simulink library "BupSimulinkLibraries"  (R2018a)
settings: Solver=VariableStepAuto  StartTime=0.0  StopTime=10.0  RelTol=1e-3
settings Model: Creator=User33  LastModifiedBy=User33

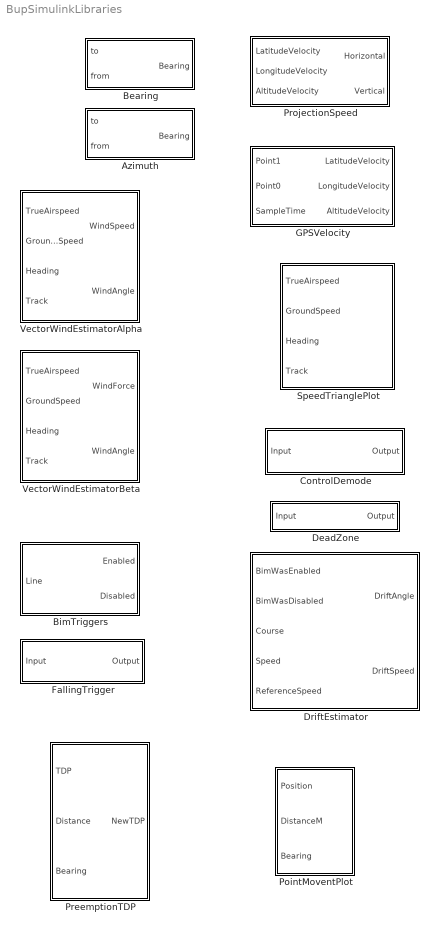
== system BupSimulinkLibraries ==
  Azimuth : Subsystem  TreatAsAtomicUnit=on
  Bearing : Subsystem  TreatAsAtomicUnit=on
  BimTriggers : Subsystem
  ControlDemode : Subsystem
  DeadZone : Subsystem
  DriftEstimator : Stateflow chart  TreatAsAtomicUnit=on
  FallingTrigger : Subsystem
  GPSVelocity : Subsystem  TreatAsAtomicUnit=on
  PointMoventPlot : Subsystem
  PreemptionTDP : Subsystem
  ProjectionSpeed : Subsystem  TreatAsAtomicUnit=on
  SpeedTrianglePlot : Subsystem
  VectorWindEstimatorAlpha : Subsystem  TreatAsAtomicUnit=on
      mask Display: image('500px-Drift_1.png');
  VectorWindEstimatorBeta : Subsystem  TreatAsAtomicUnit=on
      mask Display: image('500px-Drift_1.png');

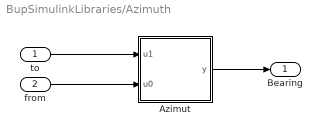
== system BupSimulinkLibraries/Azimuth ==
  to : Inport
  from : Inport  Port=2
  Azimut : MATLAB Function  TreatAsAtomicUnit=on
  Bearing : Outport
  wires:
  to/1 -> Azimut/1(u1)
  from/1 -> Azimut/2(u0)
  Azimut/1(y) -> Bearing/1

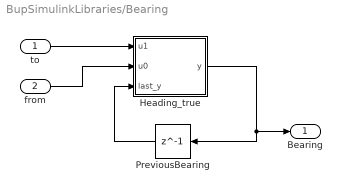
== system BupSimulinkLibraries/Bearing ==
  to : Inport
  from : Inport  Port=2
  Heading_true : MATLAB Function  TreatAsAtomicUnit=on
  PreviousBearing : Delay  DelayLength=1  InitialCondition=0
  Bearing : Outport
  wires:
  to/1 -> Heading_true/1(u1)
  Heading_true/1(y) -> PreviousBearing/1, Bearing/1
  from/1 -> Heading_true/2(u0)
  PreviousBearing/1 -> Heading_true/3(last_y)

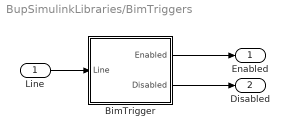
== system BupSimulinkLibraries/BimTriggers ==
  Line : Inport
  BimTrigger : Stateflow chart  TreatAsAtomicUnit=on
  Enabled : Outport
  Disabled : Outport  Port=2
  wires:
  Line/1 -> BimTrigger/1(Line)
  BimTrigger/1(Enabled) -> Enabled/1
  BimTrigger/2(Disabled) -> Disabled/1

== system BupSimulinkLibraries/ControlDemode ==
  Input : Inport
  ControlDemode : MATLAB Function  TreatAsAtomicUnit=on
  Output : Outport
  wires:
  ControlDemode/1(y) -> Output/1
  Input/1 -> ControlDemode/1(u)

== system BupSimulinkLibraries/DeadZone ==
  Input : Inport
  DeadZone : MATLAB Function  TreatAsAtomicUnit=on
  Output : Outport
  wires:
  DeadZone/1(y) -> Output/1
  Input/1 -> DeadZone/1(u)

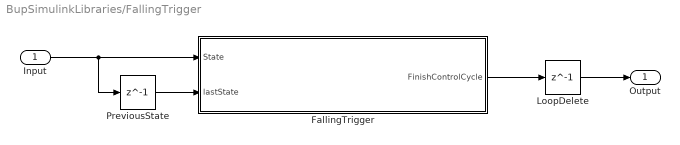
== system BupSimulinkLibraries/FallingTrigger ==
  Input : Inport
  FallingTrigger : MATLAB Function  TreatAsAtomicUnit=on
  LoopDelete : Delay  DelayLength=1
  PreviousState : Delay  DelayLength=1
  Output : Outport
  wires:
  FallingTrigger/1(FinishControlCycle) -> LoopDelete/1
  Input/1 -> PreviousState/1, FallingTrigger/1(State)
  LoopDelete/1 -> Output/1
  PreviousState/1 -> FallingTrigger/2(lastState)

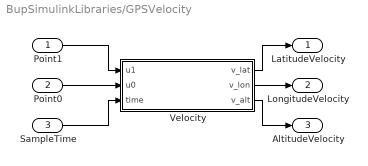
== system BupSimulinkLibraries/GPSVelocity ==
  Point1 : Inport
  Point0 : Inport  Port=2
  SampleTime : Inport  Port=3
  Velocity : MATLAB Function  TreatAsAtomicUnit=on
  LatitudeVelocity : Outport
  LongitudeVelocity : Outport  Port=2
  AltitudeVelocity : Outport  Port=3
  wires:
  Velocity/1(v_lat) -> LatitudeVelocity/1
  Point0/1 -> Velocity/2(u0)
  Point1/1 -> Velocity/1(u1)
  Velocity/3(v_alt) -> AltitudeVelocity/1
  Velocity/2(v_lon) -> LongitudeVelocity/1
  SampleTime/1 -> Velocity/3(time)

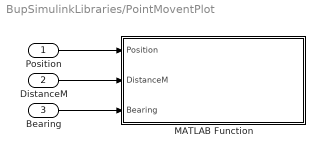
== system BupSimulinkLibraries/PointMoventPlot ==
  Position : Inport
  DistanceM : Inport  Port=2
  Bearing : Inport  Port=3
  MATLAB Function : MATLAB Function  TreatAsAtomicUnit=on
  wires:
  DistanceM/1 -> MATLAB Function/2(DistanceM)
  Bearing/1 -> MATLAB Function/3(Bearing)
  Position/1 -> MATLAB Function/1(Position)

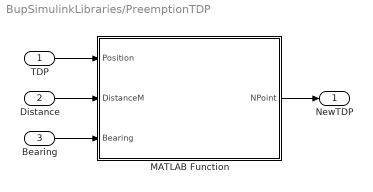
== system BupSimulinkLibraries/PreemptionTDP ==
  TDP : Inport
  Distance : Inport  Port=2
  Bearing : Inport  Port=3
  MATLAB Function : MATLAB Function  TreatAsAtomicUnit=on
  NewTDP : Outport
  wires:
  Bearing/1 -> MATLAB Function/3(Bearing)
  MATLAB Function/1(NPoint) -> NewTDP/1
  TDP/1 -> MATLAB Function/1(Position)
  Distance/1 -> MATLAB Function/2(DistanceM)

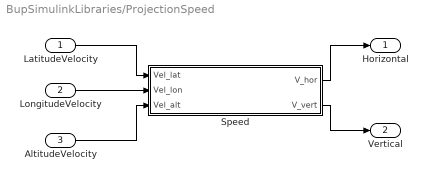
== system BupSimulinkLibraries/ProjectionSpeed ==
  LatitudeVelocity : Inport
  LongitudeVelocity : Inport  Port=2
  AltitudeVelocity : Inport  Port=3
  Speed : MATLAB Function  TreatAsAtomicUnit=on
  Horizontal : Outport
  Vertical : Outport  Port=2
  wires:
  LatitudeVelocity/1 -> Speed/1(Vel_lat)
  Speed/1(V_hor) -> Horizontal/1
  LongitudeVelocity/1 -> Speed/2(Vel_lon)
  AltitudeVelocity/1 -> Speed/3(Vel_alt)
  Speed/2(V_vert) -> Vertical/1

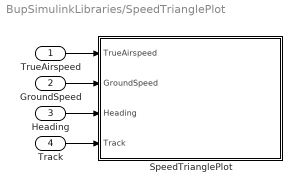
== system BupSimulinkLibraries/SpeedTrianglePlot ==
  TrueAirspeed : Inport
  GroundSpeed : Inport  Port=2
  Heading : Inport  Port=3
  Track : Inport  Port=4
  SpeedTrianglePlot : MATLAB Function  TreatAsAtomicUnit=on
  wires:
  Track/1 -> SpeedTrianglePlot/4(Track)
  Heading/1 -> SpeedTrianglePlot/3(Heading)
  GroundSpeed/1 -> SpeedTrianglePlot/2(GroundSpeed)
  TrueAirspeed/1 -> SpeedTrianglePlot/1(TrueAirspeed)

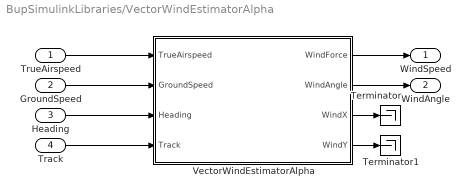
== system BupSimulinkLibraries/VectorWindEstimatorAlpha ==
  TrueAirspeed : Inport
  GroundSpeed : Inport  Port=2
  Heading : Inport  Port=3
  Track : Inport  Port=4
  Terminator : Terminator
  Terminator1 : Terminator
  VectorWindEstimatorAlpha : MATLAB Function  TreatAsAtomicUnit=on
  WindSpeed : Outport
  WindAngle : Outport  Port=2
  wires:
  VectorWindEstimatorAlpha/3(WindX) -> Terminator/1
  GroundSpeed/1 -> VectorWindEstimatorAlpha/2(GroundSpeed)
  Heading/1 -> VectorWindEstimatorAlpha/3(Heading)
  VectorWindEstimatorAlpha/1(WindForce) -> WindSpeed/1
  TrueAirspeed/1 -> VectorWindEstimatorAlpha/1(TrueAirspeed)
  Track/1 -> VectorWindEstimatorAlpha/4(Track)
  VectorWindEstimatorAlpha/4(WindY) -> Terminator1/1
  VectorWindEstimatorAlpha/2(WindAngle) -> WindAngle/1

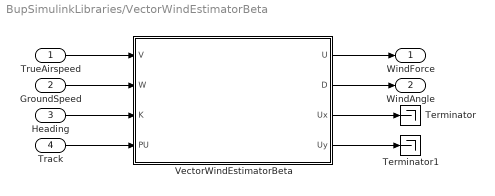
== system BupSimulinkLibraries/VectorWindEstimatorBeta ==
  TrueAirspeed : Inport
  GroundSpeed : Inport  Port=2
  Heading : Inport  Port=3
  Track : Inport  Port=4
  Terminator : Terminator
  Terminator1 : Terminator
  VectorWindEstimatorBeta : MATLAB Function  TreatAsAtomicUnit=on
  WindForce : Outport
  WindAngle : Outport  Port=2
  wires:
  VectorWindEstimatorBeta/2(D) -> WindAngle/1
  VectorWindEstimatorBeta/4(Uy) -> Terminator1/1
  VectorWindEstimatorBeta/1(U) -> WindForce/1
  Track/1 -> VectorWindEstimatorBeta/4(PU)
  Heading/1 -> VectorWindEstimatorBeta/3(K)
  GroundSpeed/1 -> VectorWindEstimatorBeta/2(W)
  VectorWindEstimatorBeta/3(Ux) -> Terminator/1
  TrueAirspeed/1 -> VectorWindEstimatorBeta/1(V)

== matlab function BupSimulinkLibraries/SpeedTrianglePlot/SpeedTrianglePlot ==
  data: TrueAirspeed input size=1; GroundSpeed input size=1; Heading input size=1; Track input size=1
%%%%%%%%%%%%%%%%%%%%%%%%%%%%%%%%%%%%%%%%%%%%%%%%%%%%%%%%%%%%%%%%%%%%%%%%%%%
%
%   Расчет и построение навигационного треугольника скоростей
%
%   Обозначения:
%   TrueAirspeed - Истинная воздушная скорость
%   GroundSpeed - Скорость относительно земли
%   Heading - Направление продольной оси
%   Track - Путевой курс
%%%%%%%%%%%%%%%%%%%%%%%%%%%%%%%%%%%%%%%%%%%%%%%%%%%%%%%%%%%%%%%%%%%%%%%%%%%
function SpeedTrianglePlot(TrueAirspeed, GroundSpeed, Heading, Track)
    %% Определяем проекции вектора воздушной скорости
    TrueAirspeedX = TrueAirspeed * cos(pi/2 - Heading);
    TrueAirspeedY = TrueAirspeed * cos(- Heading);
    %% Определяем проекции вектора путевой скорости
    GroundSpeedX = GroundSpeed * cos(pi/2 - Track);
    GroundSpeedY = GroundSpeed * cos(- Track);
    %% Определяем проекции вектора ветра
    WindX = -(TrueAirspeedX - GroundSpeedX);
    WindY = -(TrueAirspeedY - GroundSpeedY);
    %% Визуализация
    figure(55)
    plot([0 TrueAirspeedX], [0 TrueAirspeedY]);
    hold on
    plot([0 GroundSpeedX], [0 GroundSpeedY]);
    hold on
    plot([TrueAirspeedX TrueAirspeedX+WindX], [TrueAirspeedY TrueAirspeedY+WindY]);
    grid on
    hold off
    axis([-30 +30 -30 +30])
end

== matlab function BupSimulinkLibraries/Azimuth/Azimut ==
  data: u1 input size=3; u0 input size=3; y output size=1
function y = fcn(u1, u0)
% u0 - точка отсчета
% u1 - конечная точка
% la - долгота
% fi - широта
la1 = u0(2)*pi/180;
fi1 = u0(1)*pi/180;
la2 = u1(2)*pi/180;
fi2 = u1(1)*pi/180;
delta_la = la2-la1;
y = atan2(sin(delta_la)*cos(fi2), cos(fi1)*sin(fi2)-sin(fi1)*cos(fi2)*cos(delta_la));
y = rem((y + 2*pi), 2*pi);
end

== matlab function BupSimulinkLibraries/Bearing/Heading_true ==
  data: u1 input size=3; u0 input size=3; y output size=1; last_y input size=1
function y = fcn(u1, u0, last_y)
%% Высчитаем, как изменились координаты
un = u1 - u0;
d_lat = un(1);
d_lon = un(2);
%% Условие для определения кратчайшего пути с учетом переходов между
% меридианами 0 и 180 по долготе
if d_lon > 180
    d_lon = d_lon - 360;
elseif d_lon < (-180)
        d_lon = d_lon +360;
end
%% Расчет курса
un_pow1 = d_lat*d_lat;
un_pow2 = d_lon*d_lon;
if (un_pow1 < 1e-16) && (un_pow2 < 1e-16)
    y = last_y;
else
    x = acos( d_lon / (sqrt(un_pow2 + un_pow1)));
    y = acos( d_lat / (sqrt(un_pow2 + un_pow1)));
    if x > pi/2
        y = 2*pi - y;
    end
end

== matlab function BupSimulinkLibraries/ControlDemode/ControlDemode ==
  data: u input size=1; y output size=1
function y = ControlDemode(u)
    % Здесь переводим угол из диапазона [0 360]
    % в диапазон [-180 180], что позволит нам определять
    % оптимальное направление разворота (лево и право)
    y = u;
    % Если больше 180
    if y > pi
        % то это уже отрицательная полуокружность
        y = y - 2*pi;
    % Если меньше -180
    elseif (y < (-pi))
        % то это уже положительная полуокружность
        y = y + 2*pi;
    end
end

== matlab function BupSimulinkLibraries/GPSVelocity/Velocity ==
  data: u1 input size=3; v_lat output size=1; u0 input size=3; v_lon output size=1; v_alt output size=1; time input size=1
%%%%%%%%%%%%%%%%%%%%%%%%%%%%%%%%%%%%%%%%%%%%%%%%%%%%%%%%%%%%%%%%%%%%%%%%%%%
%
%   GPSPos2Speed - Определение скорости по сигналам GPS
%   u1 - Точка относительно, которой считаем перемещение (lat, lon, alt)
%   u0 - Точка до которой отладываем перемещение (lat, lon, alt)
%   time - Время между замерами координат
%
%%%%%%%%%%%%%%%%%%%%%%%%%%%%%%%%%%%%%%%%%%%%%%%%%%%%%%%%%%%%%%%%%%%%%%%%%%%
function [v_lat, v_lon, v_alt] = GPSPos2Speed(u1, u0, time)
    un = u1-u0;
    v_lat = un(1)*40000/360*1000/time;
    v_lon = un(2)*(40000/360*1000/time * cos(pi/180*u0(1)));
    v_alt = un(3);
end

== matlab function BupSimulinkLibraries/DeadZone/DeadZone ==
  data: u input size=1; y output size=1
%%%%%%%%%%%%%%%%%%%%%%%%%%%%%%%%%%%%%%%%%%%%%%%%%%%%%%%%%%%%%%%%%%%%%%%%%%%
%
%   Звено нечувствительности
%
%%%%%%%%%%%%%%%%%%%%%%%%%%%%%%%%%%%%%%%%%%%%%%%%%%%%%%%%%%%%%%%%%%%%%%%%%%%
function y = DeadZone(u)
if abs(u) < 20
    y = 0;
else
    y = u;
end
% if u > 10
%     y = 50;
% elseif u < - 10
%     y = -50;
% else
%     y = 0;
% end

== matlab function BupSimulinkLibraries/FallingTrigger/FallingTrigger ==
  data: State input size=1; FinishControlCycle output boolean size=1; lastState input size=1
function FinishControlCycle = FallingTrigger(State, lastState)
    if lastState > 0 && State <= 0
        FinishControlCycle = true;

    elseif lastState < 0 && State >= 0
        FinishControlCycle = true;

    else 
        FinishControlCycle = false;
    end
end

== matlab function BupSimulinkLibraries/ProjectionSpeed/Speed ==
  data: Vel_lat input size=1; V_hor output size=1; Vel_lon input size=1; Vel_alt input size=1; V_vert output size=1
%%%%%%%%%%%%%%%%%%%%%%%%%%%%%%%%%%%%%%%%%%%%%%%%%%%%%%%%%%%%%%%%%%%%%%%%%%%
%
%   SpeedProjections - Пересчет проекций векторов скорости по lat, lon, alt
%   в горизонтальную и вертикальную скорость полёта
%
%%%%%%%%%%%%%%%%%%%%%%%%%%%%%%%%%%%%%%%%%%%%%%%%%%%%%%%%%%%%%%%%%%%%%%%%%%%
function [V_hor, V_vert] = SpeedProjections(Vel_lat, Vel_lon, Vel_alt)
    V_hor = sqrt(Vel_lat^2 + Vel_lon^2);
    V_vert = abs(Vel_alt);
end

== stateflow chart BupSimulinkLibraries/BimTriggers/BimTrigger ==
  state Triggers
    state DisabledTrigger [parallel]
      if LastLineState > 0 && Line <=0
      Disabled = true;
      elseif LastLineState < 0 && Line >=0
      Disabled = true;
      else
      Disabled = false;
      end
      settings: executionOrder=1
    state EnabledTrigger1 [parallel]
      if LastLineState == 0 && Line > 0
      Enabled = true;
      elseif LastLineState == 0 && Line < 0
      Enabled = true;
      else
      Enabled = false;
      end
      settings: executionOrder=2
    state RemeberLastState [parallel]
      LastLineState = Line;
      settings: executionOrder=3
  data: Enabled output boolean size=1; Disabled output boolean size=1; LastLineState local double size=1 =0; Line input double size=1

== stateflow chart BupSimulinkLibraries/DriftEstimator ==
  state FixBeforeCorrection
    exit:
    RealCourse = Course;
    RealSpeed  = Speed;
  state FixAfterCorrection
    exit:
    ReferenceCourse = Course;
  state DriftSolver
    [DriftSpeed, DriftAngle] = SpeedTriangle(ReferenceSpeed, RealSpeed, ReferenceCourse, RealCourse);
    %SpeedTrianglePlot(ReferenceSpeed, RealSpeed, ReferenceCourse, RealCourse);
  (default) -> FixAfterCorrection
  FixAfterCorrection -> FixBeforeCorrection : [BimWasDisabled == 1]
  DriftSolver -> FixAfterCorrection
  FixBeforeCorrection -> DriftSolver : [BimWasEnabled == 1]
  data: BimWasEnabled input boolean size=1; BimWasDisabled input boolean size=1; Course input double size=1; Speed input double size=1; DriftAngle output double size=1; DriftSpeed output double size=1; ReferenceCourse local double size=1; RealSpeed local double size=1; RealCourse local double size=1; ReferenceSpeed input double size=1

== matlab function BupSimulinkLibraries/PreemptionTDP/MATLAB Function ==
  data: Position input double size=3; NPoint output double size=[1 3]; DistanceM input double size=1; Bearing input double size=1
%%%%%%%%%%%%%%%%%%%%%%%%%%%%%%%%%%%%%%%%%%%%%%%%%%%%%%%%%%%%%%%%%%%%%%%%%%%
%
%   PointMovement - Перемещение из точки Position на расстояние 
%   DistanceM (метры) в направлении относительно севера Bearing
%
%%%%%%%%%%%%%%%%%%%%%%%%%%%%%%%%%%%%%%%%%%%%%%%%%%%%%%%%%%%%%%%%%%%%%%%%%%%
function NPoint = PointMovement(Position, DistanceM, Bearing)
    %% Рассчитаем угловое расстояние
    AngularDistance = DistanceM/6378160;
    %% Координаты в радианы
    Lat1 = Position(1)/180*pi;
    Lon1 = Position(2)/180*pi;
    %% Получаем координаты точки перемещения
    Lat2 = asin(sin(Lat1)*cos(AngularDistance) + cos(Lat1)*sin(AngularDistance)*cos(Bearing));
    Lon2 = Lon1 + atan2(sin(Bearing)*sin(AngularDistance)*cos(Lat1), cos(AngularDistance)-sin(Lat1)*sin(Lat2));
    %% Переводим в градусы
    Lat2 = Lat2/pi*180;
    Lon2 = Lon2/pi*180;
    NPoint = [Lat2, Lon2, Position(3)];
end

== matlab function BupSimulinkLibraries/PointMoventPlot/MATLAB Function ==
  data: Position input double size=3; DistanceM input double size=1; Bearing input double size=1
%%%%%%%%%%%%%%%%%%%%%%%%%%%%%%%%%%%%%%%%%%%%%%%%%%%%%%%%%%%%%%%%%%%%%%%%%%%
%
%   PointMovementPlot - Отрисовка перемещения из точки Position на 
%   расстояние DistanceM (метры) в направлении относительно севера Bearing
%
%%%%%%%%%%%%%%%%%%%%%%%%%%%%%%%%%%%%%%%%%%%%%%%%%%%%%%%%%%%%%%%%%%%%%%%%%%%
function PointMovementPlot(Position, DistanceM, Bearing)
    %% Рассчитаем угловое расстояние
    AngularDistance = DistanceM/6378160;
    %% Координаты в радианы
    Lat1 = Position(1)/180*pi;
    Lon1 = Position(2)/180*pi;
    %% Получаем координаты точки перемещения
    Lat2 = asin(sin(Lat1)*cos(AngularDistance) + cos(Lat1)*sin(AngularDistance)*cos(Bearing));
    Lon2 = Lon1 + atan2(sin(Bearing)*sin(AngularDistance)*cos(Lat1), cos(AngularDistance)-sin(Lat1)*sin(Lat2));
    %% Переводим в градусы
    Lat2 = Lat2/pi*180;
    Lon2 = Lon2/pi*180;
    %% Визуализация
    %% Окружность
    figure(66)
    R = 100/1000*360/40000;
    plot(Position(2) + R * cos(0:0.001:2*pi), Position(1) + R * sin(0:0.001:2*pi));
    hold on
    R = 200/1000*360/40000;
    plot(Position(2) + R * cos(0:0.001:2*pi), Position(1) + R * sin(0:0.001:2*pi));
    hold on
    R = 300/1000*360/40000;
    plot(Position(2) + R * cos(0:0.001:2*pi), Position(1) + R * sin(0:0.001:2*pi));
    hold on
    R = 450/1000*360/40000;
    plot(Position(2) + R * cos(0:0.001:2*pi), Position(1) + R * sin(0:0.001:2*pi));
    hold on
    plot([Position(2), Lon2], [Position(1), Lat2]);
    grid on
    hold off
end

== matlab function BupSimulinkLibraries/VectorWindEstimatorAlpha/VectorWindEstimatorAlpha ==
  data: TrueAirspeed input size=1; WindForce output size=1; GroundSpeed input size=1; Heading input size=1; Track input size=1; WindAngle output size=1; WindX output size=1; WindY output size=1
%%%%%%%%%%%%%%%%%%%%%%%%%%%%%%%%%%%%%%%%%%%%%%%%%%%%%%%%%%%%%%%%%%%%%%%%%%%
%
%   Расчет параметров ветра по навигационному треугольнику скоростей
%
%   Обозначения:
%   TrueAirspeed - Истинная воздушная скорость
%   GroundSpeed - Скорость относительно земли
%   Heading - Направление продольной оси
%   Track - Путевой курс
%
%%%%%%%%%%%%%%%%%%%%%%%%%%%%%%%%%%%%%%%%%%%%%%%%%%%%%%%%%%%%%%%%%%%%%%%%%%%
function [WindForce, WindAngle, WindX, WindY] = SpeedTriangle(TrueAirspeed, GroundSpeed, Heading, Track)
    %% Определяем проекции вектора воздушной скорости
    TrueAirspeedX = TrueAirspeed * cos(pi/2 - Heading);
    TrueAirspeedY = TrueAirspeed * cos(- Heading);
    %% Определяем проекции вектора путевой скорости
    GroundSpeedX = GroundSpeed * cos(pi/2 - Track);
    GroundSpeedY = GroundSpeed * cos(- Track);
    %% Определяем проекции вектора ветра
    WindX = -(TrueAirspeedX - GroundSpeedX);
    WindY = -(TrueAirspeedY - GroundSpeedY);
    %% Определяем модуль вектора ветра
    powY = WindY*WindY;
    powX = WindX*WindX;
    WindForce = sqrt(powX + powY);
    %% Расчет направления ветра
    %% 
    if (powX < 1e-16) && (powY < 1e-16)
        y = 0;
    else
        x = acos( WindX / (sqrt(powX + powY)));
        y = acos( WindY / (sqrt(powX + powY)));
        if x > 1.5708
            y = 6.28319 - y;
        end
    end
    WindAngle = y;
end

== matlab function BupSimulinkLibraries/VectorWindEstimatorBeta/VectorWindEstimatorBeta ==
  data: V input size=1; U output size=1; W input size=1; K input size=1; PU input size=1; D output size=1; Ux output size=1; Uy output size=1
%%%%%%%%%%%%%%%%%%%%%%%%%%%%%%%%%%%%%%%%%%%%%%%%%%%%%%%%%%%%%%%%%%%%%%%%%%%
%
%    Рассчет параметров ветра по навигационному треугольнику скоростей
%
%   Обозначения:
%   W - Путевая скорость
%   V - Воздушная скорость
%   K - Курс
%   PU - Путевой курс
%   U - Скорость ветра
%   D - Направление ветра
%
%%%%%%%%%%%%%%%%%%%%%%%%%%%%%%%%%%%%%%%%%%%%%%%%%%%%%%%%%%%%%%%%%%%%%%%%%%%
function [U, D, Ux, Uy] = SpeedTriangle2(V, W, K, PU)
    Ux = 0;
    Uy = 0;
    %% Определяем угол сноса
    US = PU - K;
    %% Курсовой угол ветра
    AC = W * sin(US); % вспомогательная сторона треугольника
    %% Определяем курсовой угол ветра
    %KUV = atan2(AC,W-V); - это приближение можно использовать для малых углов
    KUV = atan2(AC,W*cos(US)-V);
    %% Определяем модуль вектора ветра
    U = AC/sin(KUV);
    %% Определяем абсолютный угол ветра относительно севера
    D = K + KUV;
    % Разрешаем ему быть всегда только положительным
    if D > 2*pi 
        D = D - 2*pi;
    elseif D < 0
        D = D + 2*pi;
    end
end
